simulink model "Basic_scheme"  (R2018a)
settings: Solver=VariableStepAuto  StartTime=0.0  StopTime=0.2  RelTol=1e-3
libraries: dsparch4 x6, commdigbbndpm3 x3, commrandsrc2 x1, dspsigops x1
settings Model: Creator=1  LastModifiedBy=1

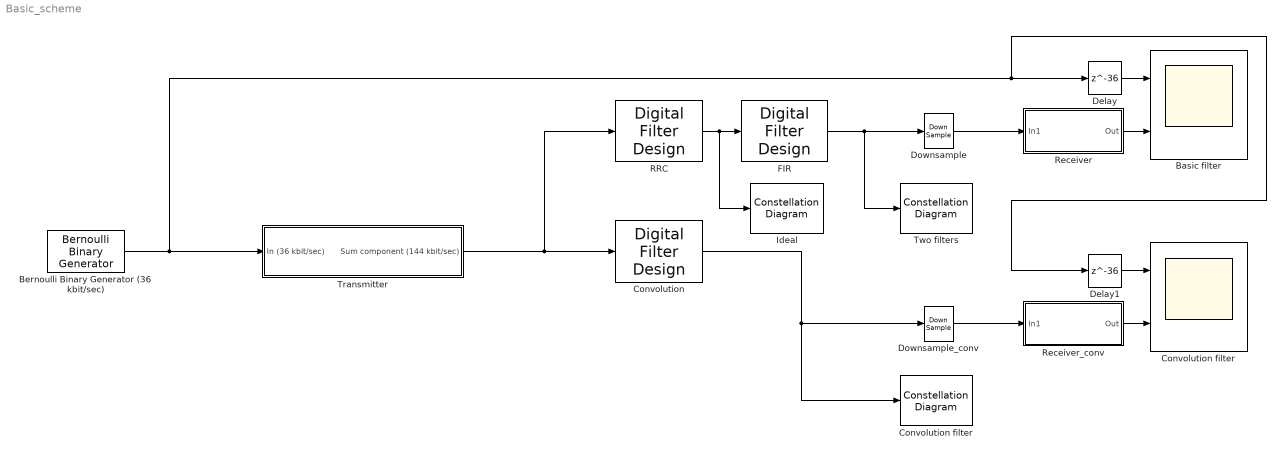
== system Basic_scheme ==
  Basic filter : Scope  NumInputPorts=2
  "Bernoulli Binary Generator (36 kbit/sec) " : commrandsrc2/Bernoulli Binary Generator  P=0.5  seed=11  Ts=1/(36*10^3)  frameBased=off  sampPerFrame=1  orient=off  outDataType=double
  Convolution : dsparch4/Digital Filter Design  mwdsp_browser_bugfix_var=off
  Convolution filter : Scope  NumInputPorts=2
  "Convolution filter " : ConstellationDiagram  Tag=ScatterPlot
  Delay : Delay  DelayLength=36
  Delay1 : Delay  DelayLength=36
  Downsample : DownSample  N=8  RateOptions=Allow multirate processing
  Downsample_conv : DownSample  N=8  RateOptions=Allow multirate processing
  FIR : dsparch4/Digital Filter Design  mwdsp_browser_bugfix_var=off
  Ideal : ConstellationDiagram  Tag=ScatterPlot
  RRC : dsparch4/Digital Filter Design  mwdsp_browser_bugfix_var=off
  Receiver : Subsystem
  Receiver_conv : Subsystem
  "Transmitter " : Subsystem
  Two filters : ConstellationDiagram  Tag=ScatterPlot
  wires:
  "Bernoulli Binary Generator (36 kbit/sec) "/1 -> Delay1/1, Delay/1, "Transmitter "/1(In (36 kbit/sec))
  Receiver/1(Out) -> Basic filter/2
  Delay/1 -> Basic filter/1
  RRC/1 -> Ideal/1, FIR/1
  FIR/1 -> Downsample/1, Two filters/1
  Downsample/1 -> Receiver/1(In1)
  Receiver_conv/1(Out) -> Convolution filter/2
  Delay1/1 -> Convolution filter/1
  Convolution/1 -> Downsample_conv/1, "Convolution filter "/1
  Downsample_conv/1 -> Receiver_conv/1(In1)
  "Transmitter "/1(Sum component (144 kbit/sec)) -> RRC/1, Convolution/1

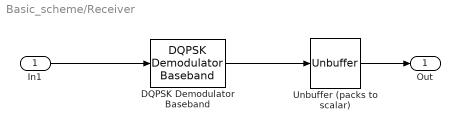
== system Basic_scheme/Receiver ==
  In1 : Inport
  DQPSK Demodulator Baseband : commdigbbndpm3/DQPSK Demodulator Baseband  OutType=Bit  Dec=Gray  Ph=pi/4  outDtype1=Inherit via internal rule  outDtype2=Inherit via internal rule
      settings: SourceProductName=Communications System Toolbox  SourceProductBaseCode=CM
  Unbuffer (packs to scalar) : Unbuffer
  Out : Outport
  wires:
  DQPSK Demodulator Baseband/1 -> Unbuffer (packs to scalar)/1
  Unbuffer (packs to scalar)/1 -> Out/1
  In1/1 -> DQPSK Demodulator Baseband/1

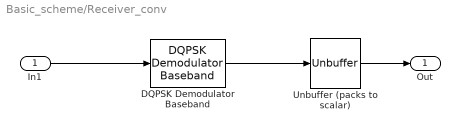
== system Basic_scheme/Receiver_conv ==
  In1 : Inport
  DQPSK Demodulator Baseband : commdigbbndpm3/DQPSK Demodulator Baseband  OutType=Bit  Dec=Gray  Ph=pi/4  outDtype1=Inherit via internal rule  outDtype2=Inherit via internal rule
      settings: SourceProductName=Communications System Toolbox  SourceProductBaseCode=CM
  Unbuffer (packs to scalar) : Unbuffer
  Out : Outport
  wires:
  DQPSK Demodulator Baseband/1 -> Unbuffer (packs to scalar)/1
  Unbuffer (packs to scalar)/1 -> Out/1
  In1/1 -> DQPSK Demodulator Baseband/1

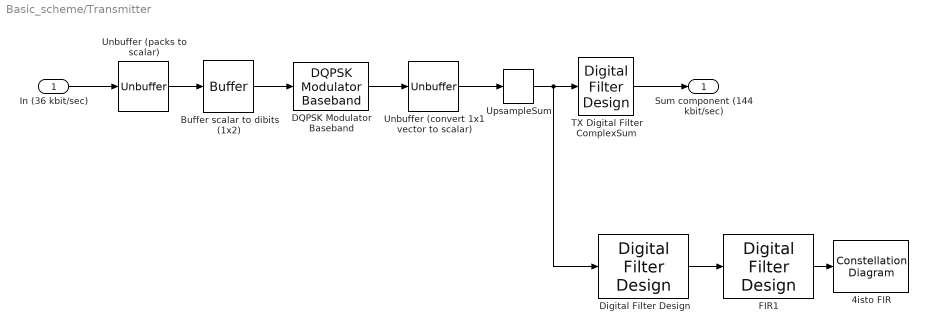
== system Basic_scheme/Transmitter  ==
  In (36 kbit/sec) : Inport  SampleTime=1/(36*10^3)
  4isto FIR : ConstellationDiagram  Tag=ScatterPlot
  "Buffer scalar to dibits (1x2) " : Buffer  N=2
  DQPSK Modulator Baseband : commdigbbndpm3/DQPSK Modulator Baseband  InType=Bit  Enc=Gray  Ph=pi/4  outDtype=double
      settings: SourceProductName=Communications System Toolbox  SourceProductBaseCode=CM
  Digital Filter Design : dsparch4/Digital Filter Design  mwdsp_browser_bugfix_var=off
  FIR1 : dsparch4/Digital Filter Design  mwdsp_browser_bugfix_var=off
  TX Digital Filter ComplexSum : dsparch4/Digital Filter Design  mwdsp_browser_bugfix_var=off
  "Unbuffer (convert 1x1 vector to scalar) " : Unbuffer
  Unbuffer (packs to scalar) : Unbuffer
  UpsampleSum : dspsigops/Upsample  N=8  phase=0  RateOptions=Allow multirate processing  ic=0  mode=Unused parameter value
  Sum component (144 kbit/sec) : Outport  OutDataTypeStr=double  SampleTime=1/(144*(10^3))
      settings: SignalType=complex
  wires:
  In (36 kbit/sec)/1 -> Unbuffer (packs to scalar)/1
  Unbuffer (packs to scalar)/1 -> "Buffer scalar to dibits (1x2) "/1
  "Buffer scalar to dibits (1x2) "/1 -> DQPSK Modulator Baseband/1
  "Unbuffer (convert 1x1 vector to scalar) "/1 -> UpsampleSum/1
  DQPSK Modulator Baseband/1 -> "Unbuffer (convert 1x1 vector to scalar) "/1
  UpsampleSum/1 -> Digital Filter Design/1, TX Digital Filter ComplexSum/1
  TX Digital Filter ComplexSum/1 -> Sum component (144 kbit/sec)/1
  FIR1/1 -> 4isto FIR/1
  Digital Filter Design/1 -> FIR1/1
